simulink model "Pressure_Drop_StaticHeight_example"  (Simulink 7.6)
settings: Solver=ode45  StartTime=0.0  StopTime=10.0  RelTol=1e-3
libraries: carnot x2
settings Model: Creator=drhf  LastModifiedBy=drhf

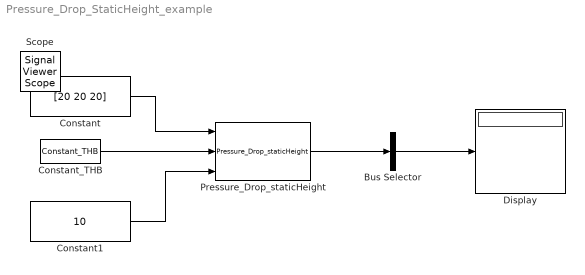
== system Pressure_Drop_StaticHeight_example ==
  Bus Selector : BusSelector  OutputSignals=Pressure,GeodeticHeight  OutputAsBus=on
  Constant : Constant  Value=[20 20 20]
  Constant1 : Constant  Value=10
  Constant_THB : carnot/Source/Simple/Constant_THB  SystemSampleTime=-1  t=40  mdot=0*100/3600  p=2e5  mID=Full Pressure Drop with Static Height  fluid=water  mix=0  dia=0.02  hgt=0
  Display : Display
  Pressure_Drop_staticHeight : carnot/Basic/Pressure_Drop/Pressure_Drop_staticHeight  SystemSampleTime=-1
  Scope : SignalViewerScope  IOType=viewer  RefreshTime=0.035000
  wires:
  Constant_THB/1 -> Pressure_Drop_staticHeight/2
  Constant/1 -> Pressure_Drop_staticHeight/1
  Pressure_Drop_staticHeight/1 -> Bus Selector/1
  Bus Selector/1 -> Display/1
  Constant1/1 -> Pressure_Drop_staticHeight/3
